simulink model "P2j"  (R2021b)
settings: Solver=FixedStepAuto  StartTime=0.0  StopTime=20  RelTol=1e-3  EnableMultiTasking=on
libraries: arduinolib x2
settings Model: ExtModeTrigDuration=2  Creator=KEMPIS VILLAMIL  LastModifiedBy=parra
settings OptimizationCC: EnhancedBackFolding=on  PassReuseOutputArgsAs=Individual arguments  ZeroExternalMemoryAtStartup=off  ZeroInternalMemoryAtStartup=off  MaxStackSize=64  OptimizeBlockOrder=speed  DifferentSizesBufferReuse=on  OptimizationCustomize=off  EfficientTunableParamExpr=on
settings DebuggingCC: ParameterTunabilityLossMsg=error  UnconnectedInputMsg=none  UnconnectedOutputMsg=none  UnconnectedLineMsg=none
settings HardwareCC: ProdBitPerInt=16  ProdBitPerPointer=16  ProdBitPerSizeT=16  ProdBitPerPtrDiffT=16  ProdLargestAtomicFloat=None  ProdWordSize=8  ProdHWDeviceType=Atmel->AVR
settings ModelReferenceCC: EnableRefExpFcnMdlSchedulingChecks=off
settings SFSimCC: MATLABDynamicMemAlloc=off
settings RTWCC: Description=Embedded Coder  SystemTargetFile=ert.tlc  HardwareBoard=Arduino Uno  TemplateMakefile=ert_default_tmf  Toolchain=Arduino AVR  BuildConfiguration=Faster Runs  DLArmComputeVersion=20.02.1
settings CodeAppCC: ForceParamTrailComments=on  IgnoreCustomStorageClasses=off  OperatorAnnotations=on  SimulinkDataObjDesc=on  SFDataObjDesc=on  InsertBlockDesc=on
settings ERTTargetCC: SupportContinuousTime=on  SupportVariableSizeSignals=on  ExtModeTransport=3  ExtModeStaticAlloc=on  ExtModeStaticAllocSize=250  ExtModeMexFile=ext_xcp  ExtModeIntrfLevel=Level2 - Open

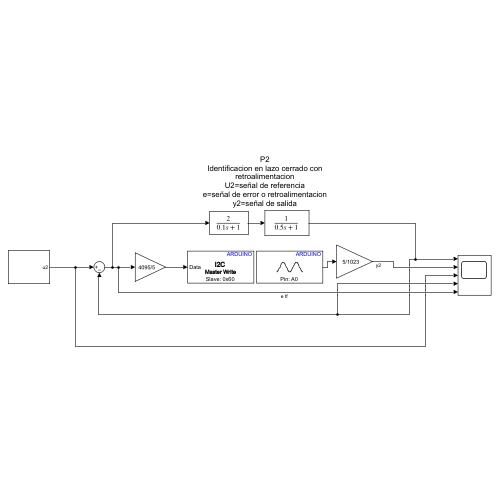
[thumbnail: Simulink's stored preview of the top-level diagram]
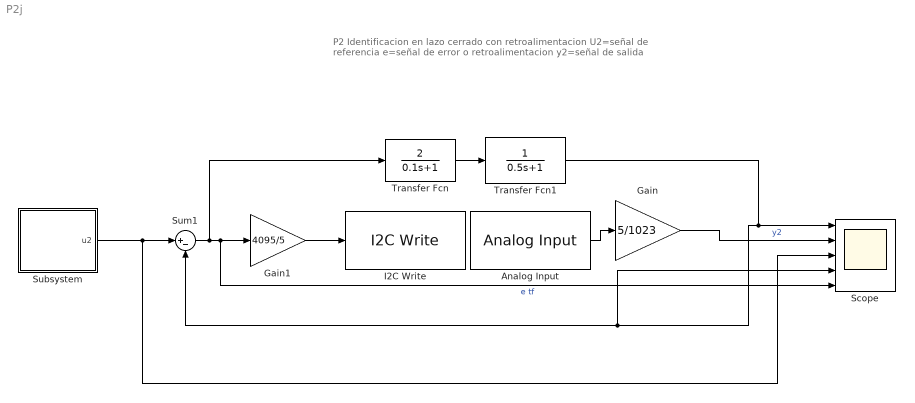
== system P2j ==
  note: P2
      | Identificacion en lazo cerrado con retroalimentacion
      | U2=señal de referencia
      | e=señal de error o retroalimentacion
      | y2=señal de salida
  Analog Input : arduinolib/Analog Input  pinNumber=0  ReadResultsOnly=off  ConversionTriggerSource=Software  ExternalTriggerType=uint32( 0 )  OutputDataType=uint16  EnableConversionCompleteNotify=off  EnableOuputStatus=off  SampleTime=0.01  blockPlatform=arduino
  Gain : Gain  Gain=5/1023
  Gain1 : Gain  Gain=4095/5  OutDataTypeStr=uint16
  I2C Write : arduinolib/I2C Write  I2CModule=0  Mode=Master  SlaveAddress=96  SlaveByteOrder=BigEndian  Direction=Transmitter  RegisterAddressMode=off  RegisterAddress=0  SlaveDataType=uint8  DataLength=1  NoAck=off  RepeatedStart=off  OutputStatus=off  blockPlatform=ARDUINO
      settings: SourceProductBaseCode=ARDUINO
  Scope : Scope  NumInputPorts=5
  Subsystem : Subsystem
  Sum1 : Sum  Inputs=|+-
  Transfer Fcn : TransferFcn  Numerator=[2]  Denominator=[0.1 1]
  Transfer Fcn1 : TransferFcn  Denominator=[0.5 1]
  wires:
  Gain1/1 -> I2C Write/1
  Gain/1 -> Scope/2  "y2"
  Analog Input/1 -> Gain/1
  Sum1/1 -> Transfer Fcn/1, Scope/5, Gain1/1  "e tf"
  Subsystem/1(u2) -> Scope/3, Sum1/1
  Transfer Fcn/1 -> Transfer Fcn1/1
  Transfer Fcn1/1 -> Scope/1, Scope/4, Sum1/2

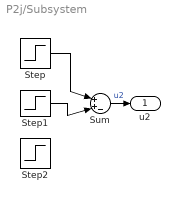
== system P2j/Subsystem ==
  Step : Step  Time=10  Before=0.5  SampleTime=0.01
  Step1 : Step  Time=13  Before=1  After=1.5  SampleTime=0.01
  Step2 : Step  Time=16  Before=1  After=1.5  SampleTime=0.01
  Sum : Sum  Inputs=|++-
  u2 : Outport
  wires:
  Step1/1 -> Sum/2
  Step/1 -> Sum/1
  Sum/1 -> u2/1  "u2"
